simulink model "TrajectoryFollowVehicleWith14DoF_"  (R2024b)
settings: Solver=VariableStepAuto  StartTime=0  StopTime=14  FixedStep=timeStep  RelTol=1e-3
PreLoadFcn:
  | useDynamicsStanley = false; %Simulink model to move according to the scenario trajectory.
  | vehicleVariant = "3DOF";
PostLoadFcn:
  | load(fullfile(matlabroot,'toolbox','driving','drivingdata','rrScenarioSimTypes.mat'));
  | helperSLTrajectoryFollowerWithRRScenarioSetup();
  | hegihtMap = "flat";
  | if isfile("pathFollowingUtil/gridMap_groundHeight_RT.mat")
  |     load("gridMap_groundHeight_RT.mat");
  | end
  | % if exist("z_2DTable", "var") && exist("xBreakPts", "var") && exist("yBreakPts", "var")
  | %     hegihtMap = "2DMap";
  | % end
  | % if isfile("CRG/crgRoad.crg")
  | %     crgData = crg_read('CRG/crgRoad.crg');
  | % end
InitFcn:
  | if ~exist("slBus42", "var")
  |     load("Bus_VehFdbk.mat");
  | end
StartFcn:
  | % set_param(bdroot, 'Profile', 'on');
StopFcn:
  | % set_param(bdroot, 'Profile', 'off');
  | % slprofreport(bdroot, 'report14DoF.html');
undefined symbols (not defined in the file or in its folder): control_timeStep, Defined, Ego, egoInitialPose, egoInitialPoseCG, egoInitialPoseRear, InitVehicle, Lane, lr, m, magnitude, max_dc, n, Pose, RRtimeStep, SceneData, steerGear, tau, tau2, timeStep, User, VehicleData, Velocity, X, xBreakPts, Y, yBreakPts, Z, z_2DTable
libraries: sm_lib x40, nesl_utility x25, simulink_extras x12, sm_vehicle_utilities_lib x7, roadrunnerscenario x6, drivingvehiclecontroller x4, mpcadaslib x1, autolibshared x1
(part 3 of 3)

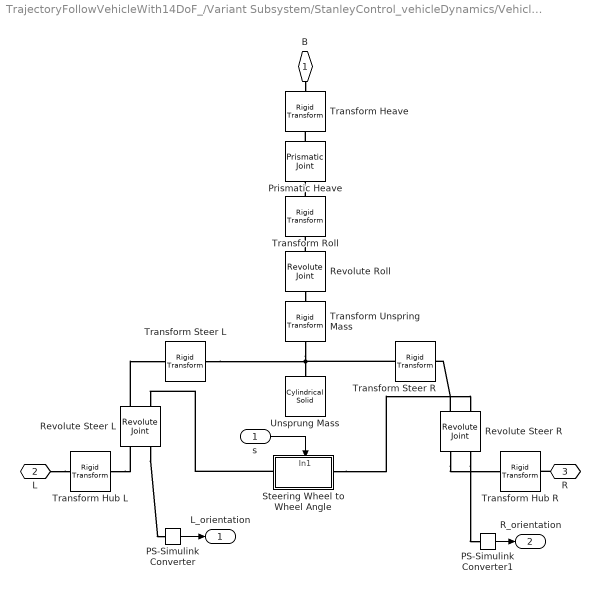
== system TrajectoryFollowVehicleWith14DoF_/Variant Subsystem/StanleyControl_vehicleDynamics/Vehicle Dynamics1/Vehicle Dynamics Multibody/Vehicle/Suspension Front ==
  s : Inport
  PS-Simulink Converter : nesl_utility/PS-Simulink Converter  PhysicalDomain=network_engine_domain  SubClassName=ps_output  LeftPortType=input  RightPortType=output  PseudoPeriodic=off  Frequencies=[]  VectorFormat=inherit  Unit=inherit  AffineConversion=off
  PS-Simulink Converter1 : nesl_utility/PS-Simulink Converter  PhysicalDomain=network_engine_domain  SubClassName=ps_output  LeftPortType=input  RightPortType=output  PseudoPeriodic=off  Frequencies=[]  VectorFormat=inherit  Unit=inherit  AffineConversion=off
  Prismatic Heave : sm_lib/Joints/Prismatic Joint  JointMode=Normal  CompositeWrenchDir=FollowerOnBase  CompositeWrenchFrame=BaseFrame  SenseConstraintForce=off  SenseConstraintTorque=off  SenseTotalForce=off  SenseTotalTorque=off  PositionTargetSpecify=off  PositionTargetPriority=High  PositionTargetValue=0  PositionTargetValueUnits=m  VelocityTargetSpecify=off  VelocityTargetPriority=High  VelocityTargetValue=0  VelocityTargetValueUnits=m/s  EquilibriumPosition=xEqHeave  EquilibriumPositionUnits=m  SpringStiffness=kHeave  SpringStiffnessUnits=N/m  DampingCoefficient=dHeave  DampingCoefficientUnits=N/(m/s)  LowerLimitSpecify=off  LowerLimitBound=-1  LowerLimitBoundUnits=m  LowerLimitStiffness=1e6  LowerLimitStiffnessUnits=N/m  LowerLimitDamping=1e3  LowerLimitDampingUnits=N/(m/s)  LowerLimitTransitionRegionWidth=1e-4  LowerLimitTransitionRegionWidthUnits=m  UpperLimitSpecify=off  UpperLimitBound=1  UpperLimitBoundUnits=m  UpperLimitStiffness=1e6  UpperLimitStiffnessUnits=N/m  UpperLimitDamping=1e3  UpperLimitDampingUnits=N/(m/s)  UpperLimitTransitionRegionWidth=1e-4  UpperLimitTransitionRegionWidthUnits=m  TorqueActuationMode=NoTorque  MotionActuationMode=ComputedMotion  SensePosition=off  SenseVelocity=off  SenseAcceleration=off  SenseTorqueForce=off  SenseLowerLimitTorqueForce=off  SenseUpperLimitTorqueForce=off
  Revolute Steer L : sm_lib/Joints/Revolute Joint  JointMode=Normal  CompositeWrenchDir=FollowerOnBase  CompositeWrenchFrame=BaseFrame  SenseConstraintForce=off  SenseConstraintTorque=off  SenseTotalForce=off  SenseTotalTorque=off  PositionTargetSpecify=off  PositionTargetPriority=High  PositionTargetValue=0  PositionTargetValueUnits=deg  VelocityTargetSpecify=off  VelocityTargetPriority=High  VelocityTargetValue=66  VelocityTargetValueUnits=rad/s  EquilibriumPosition=0  EquilibriumPositionUnits=rad  SpringStiffness=0  SpringStiffnessUnits=N*m/rad  DampingCoefficient=0  DampingCoefficientUnits=N*m/(rad/s)  LowerLimitSpecify=off  LowerLimitBound=-90  LowerLimitBoundUnits=deg  LowerLimitStiffness=1e4  LowerLimitStiffnessUnits=N*m/deg  LowerLimitDamping=10  LowerLimitDampingUnits=N*m/(deg/s)  LowerLimitTransitionRegionWidth=0.1  LowerLimitTransitionRegionWidthUnits=deg  UpperLimitSpecify=off  UpperLimitBound=90  UpperLimitBoundUnits=deg  UpperLimitStiffness=1e4  UpperLimitStiffnessUnits=N*m/deg  UpperLimitDamping=10  UpperLimitDampingUnits=N*m/(deg/s)  UpperLimitTransitionRegionWidth=0.1  UpperLimitTransitionRegionWidthUnits=deg  TorqueActuationMode=ComputedTorque  MotionActuationMode=InputMotion  SensePosition=on  SenseVelocity=off  SenseAcceleration=off  SenseTorqueForce=off  SenseLowerLimitTorqueForce=off  SenseUpperLimitTorqueForce=off
  Revolute Steer R : sm_lib/Joints/Revolute Joint  JointMode=Normal  CompositeWrenchDir=FollowerOnBase  CompositeWrenchFrame=BaseFrame  SenseConstraintForce=off  SenseConstraintTorque=off  SenseTotalForce=off  SenseTotalTorque=off  PositionTargetSpecify=off  PositionTargetPriority=High  PositionTargetValue=0  PositionTargetValueUnits=deg  VelocityTargetSpecify=off  VelocityTargetPriority=High  VelocityTargetValue=66  VelocityTargetValueUnits=rad/s  EquilibriumPosition=0  EquilibriumPositionUnits=rad  SpringStiffness=0  SpringStiffnessUnits=N*m/rad  DampingCoefficient=0  DampingCoefficientUnits=N*m/(rad/s)  LowerLimitSpecify=off  LowerLimitBound=-90  LowerLimitBoundUnits=deg  LowerLimitStiffness=1e4  LowerLimitStiffnessUnits=N*m/deg  LowerLimitDamping=10  LowerLimitDampingUnits=N*m/(deg/s)  LowerLimitTransitionRegionWidth=0.1  LowerLimitTransitionRegionWidthUnits=deg  UpperLimitSpecify=off  UpperLimitBound=90  UpperLimitBoundUnits=deg  UpperLimitStiffness=1e4  UpperLimitStiffnessUnits=N*m/deg  UpperLimitDamping=10  UpperLimitDampingUnits=N*m/(deg/s)  UpperLimitTransitionRegionWidth=0.1  UpperLimitTransitionRegionWidthUnits=deg  TorqueActuationMode=ComputedTorque  MotionActuationMode=InputMotion  SensePosition=on  SenseVelocity=off  SenseAcceleration=off  SenseTorqueForce=off  SenseLowerLimitTorqueForce=off  SenseUpperLimitTorqueForce=off
  Revolute Roll : sm_lib/Joints/Revolute Joint  JointMode=Normal  CompositeWrenchDir=FollowerOnBase  CompositeWrenchFrame=BaseFrame  SenseConstraintForce=off  SenseConstraintTorque=off  SenseTotalForce=off  SenseTotalTorque=off  PositionTargetSpecify=off  PositionTargetPriority=High  PositionTargetValue=0  PositionTargetValueUnits=deg  VelocityTargetSpecify=off  VelocityTargetPriority=High  VelocityTargetValue=0  VelocityTargetValueUnits=deg/s  EquilibriumPosition=aEqRoll  EquilibriumPositionUnits=rad  SpringStiffness=kRoll  SpringStiffnessUnits=N*m/rad  DampingCoefficient=dRoll  DampingCoefficientUnits=N*m/(rad/s)  LowerLimitSpecify=off  LowerLimitBound=-90  LowerLimitBoundUnits=deg  LowerLimitStiffness=1e4  LowerLimitStiffnessUnits=N*m/deg  LowerLimitDamping=10  LowerLimitDampingUnits=N*m/(deg/s)  LowerLimitTransitionRegionWidth=0.1  LowerLimitTransitionRegionWidthUnits=deg  UpperLimitSpecify=off  UpperLimitBound=90  UpperLimitBoundUnits=deg  UpperLimitStiffness=1e4  UpperLimitStiffnessUnits=N*m/deg  UpperLimitDamping=10  UpperLimitDampingUnits=N*m/(deg/s)  UpperLimitTransitionRegionWidth=0.1  UpperLimitTransitionRegionWidthUnits=deg  TorqueActuationMode=NoTorque  MotionActuationMode=ComputedMotion  SensePosition=off  SenseVelocity=off  SenseAcceleration=off  SenseTorqueForce=off  SenseLowerLimitTorqueForce=off  SenseUpperLimitTorqueForce=off
  Steering Wheel to Wheel Angle : Subsystem
      settings: PortSchema="{\"entries\":[{\"content\":{\"sides\":[{\"content\":{\"connectorIds\":[\"LConn1\"]},\"type\":\"ConnectorPlacement.EquallySpacedRectSide\",\"uuid\":\"65a6d75a-79bf-476b-9435-04bcf6c2ef18\"},{\"content\":{\"connectorIds\":[\"RConn1\"],\"side\":\"RIGHT\"},\"type\":\"ConnectorPlacement.EquallySpacedRectSide\",\"uuid\":\"4d91bb65-021e-4e19-8917-9509e9fd2683\"},{\"content\":{\"connectorIds\":[\"In1\"],\"side\":\"TOP\"},\"type\":\"ConnectorPlacement.EquallySpacedRectSide\",\"uuid\":\"f7aac0ed-f2d6-4a01-9627-e78393360ed0\"}]},\"type\":\"ConnectorPlacement.EquallySpacedConnector\",\"uuid\":\"6c2d29d9-099e-4079-9b4f-de2c4ae6c2a7\"}],\"packageUris\":[\"http://schema.mathworks.com/mf0/Connector/R2020b\"],\"version\":\"1.0\"}"
  Transform Heave : sm_lib/Frames and Transforms/Rigid Transform  RotationMethod=None  FollAlignAxisA=+X  BaseAlignAxisA=+Y  FollAlignAxisB=+Y  BaseAlignAxisB=+Z  RotationStandardAxis=+Z  RotationAngle=0.0  RotationAngleUnits=deg  RotationArbitraryAxis=[0 0 1]  RotationSequenceAxes=FollowerAxes  RotationSequence=XYX  RotationSequenceAngles=[0 0 0]  RotationSequenceAnglesUnits=deg  RotationMatrix=[1 0 0; 0 1 0; 0 0 1]  Quaternion=[1 0 0 0]  TranslationMethod=StandardAxis  TranslationCartesianOffset=[0 0 0]  TranslationCartesianOffsetUnits=m  TranslationStandardAxis=+Z  TranslationStandardOffset=zHeave  TranslationStandardOffsetUnits=m  TranslationROffset=0  TranslationROffsetUnits=m  TranslationThetaOffset=0  TranslationThetaOffsetUnits=deg  TranslationZOffset=0  TranslationZOffsetUnits=m
  Transform Hub L : sm_lib/Frames and Transforms/Rigid Transform  RotationMethod=StandardAxis  FollAlignAxisA=+X  BaseAlignAxisA=+Y  FollAlignAxisB=+Y  BaseAlignAxisB=+Z  RotationStandardAxis=-Y  RotationAngle=90  RotationAngleUnits=deg  RotationArbitraryAxis=[0 0 1]  RotationSequenceAxes=FollowerAxes  RotationSequence=XYX  RotationSequenceAngles=[0 0 0]  RotationSequenceAnglesUnits=deg  RotationMatrix=[1 0 0; 0 1 0; 0 0 1]  Quaternion=[1 0 0 0]  TranslationMethod=None  TranslationCartesianOffset=[0 0 0]  TranslationCartesianOffsetUnits=m  TranslationStandardAxis=+Z  TranslationStandardOffset=0  TranslationStandardOffsetUnits=m  TranslationROffset=0  TranslationROffsetUnits=m  TranslationThetaOffset=0  TranslationThetaOffsetUnits=deg  TranslationZOffset=0  TranslationZOffsetUnits=m
  Transform Hub R : sm_lib/Frames and Transforms/Rigid Transform  RotationMethod=StandardAxis  FollAlignAxisA=+X  BaseAlignAxisA=+Y  FollAlignAxisB=+Y  BaseAlignAxisB=+Z  RotationStandardAxis=-Y  RotationAngle=90  RotationAngleUnits=deg  RotationArbitraryAxis=[0 0 1]  RotationSequenceAxes=FollowerAxes  RotationSequence=XYX  RotationSequenceAngles=[0 0 0]  RotationSequenceAnglesUnits=deg  RotationMatrix=[1 0 0; 0 1 0; 0 0 1]  Quaternion=[1 0 0 0]  TranslationMethod=None  TranslationCartesianOffset=[0 0 0]  TranslationCartesianOffsetUnits=m  TranslationStandardAxis=+Z  TranslationStandardOffset=0  TranslationStandardOffsetUnits=m  TranslationROffset=0  TranslationROffsetUnits=m  TranslationThetaOffset=0  TranslationThetaOffsetUnits=deg  TranslationZOffset=0  TranslationZOffsetUnits=m
  Transform Roll : sm_lib/Frames and Transforms/Rigid Transform  RotationMethod=RotationSequence  FollAlignAxisA=+X  BaseAlignAxisA=+Y  FollAlignAxisB=+Y  BaseAlignAxisB=+Z  RotationStandardAxis=+Y  RotationAngle=90  RotationAngleUnits=deg  RotationArbitraryAxis=[0 0 1]  RotationSequenceAxes=FollowerAxes  RotationSequence=YZY  RotationSequenceAngles=[90 180 0]  RotationSequenceAnglesUnits=deg  RotationMatrix=[1 0 0; 0 1 0; 0 0 1]  Quaternion=[1 0 0 0]  TranslationMethod=StandardAxis  TranslationCartesianOffset=[0 0 0]  TranslationCartesianOffsetUnits=m  TranslationStandardAxis=+Z  TranslationStandardOffset=-zHeave+zRoll  TranslationStandardOffsetUnits=m  TranslationROffset=0  TranslationROffsetUnits=m  TranslationThetaOffset=0  TranslationThetaOffsetUnits=deg  TranslationZOffset=0  TranslationZOffsetUnits=m
  Transform Steer L : sm_lib/Frames and Transforms/Rigid Transform  RotationMethod=StandardAxis  FollAlignAxisA=+X  BaseAlignAxisA=+Y  FollAlignAxisB=+Y  BaseAlignAxisB=+Z  RotationStandardAxis=+Y  RotationAngle=90  RotationAngleUnits=deg  RotationArbitraryAxis=[0 0 1]  RotationSequenceAxes=FollowerAxes  RotationSequence=XYX  RotationSequenceAngles=[0 0 0]  RotationSequenceAnglesUnits=deg  RotationMatrix=[1 0 0; 0 1 0; 0 0 1]  Quaternion=[1 0 0 0]  TranslationMethod=Cartesian  TranslationCartesianOffset=[-zUnsprungMass+zHub 0 yTrack/2]  TranslationCartesianOffsetUnits=m  TranslationStandardAxis=+Z  TranslationStandardOffset=0  TranslationStandardOffsetUnits=m  TranslationROffset=0  TranslationROffsetUnits=m  TranslationThetaOffset=0  TranslationThetaOffsetUnits=deg  TranslationZOffset=0  TranslationZOffsetUnits=m
  Transform Steer R : sm_lib/Frames and Transforms/Rigid Transform  RotationMethod=StandardAxis  FollAlignAxisA=+X  BaseAlignAxisA=+Y  FollAlignAxisB=+Y  BaseAlignAxisB=+Z  RotationStandardAxis=+Y  RotationAngle=90  RotationAngleUnits=deg  RotationArbitraryAxis=[0 0 1]  RotationSequenceAxes=FollowerAxes  RotationSequence=XYX  RotationSequenceAngles=[0 0 0]  RotationSequenceAnglesUnits=deg  RotationMatrix=[1 0 0; 0 1 0; 0 0 1]  Quaternion=[1 0 0 0]  TranslationMethod=Cartesian  TranslationCartesianOffset=[-zUnsprungMass+zHub 0 -yTrack/2]  TranslationCartesianOffsetUnits=m  TranslationStandardAxis=+Z  TranslationStandardOffset=0  TranslationStandardOffsetUnits=m  TranslationROffset=0  TranslationROffsetUnits=m  TranslationThetaOffset=0  TranslationThetaOffsetUnits=deg  TranslationZOffset=0  TranslationZOffsetUnits=m
  Transform Unspring Mass : sm_lib/Frames and Transforms/Rigid Transform  RotationMethod=StandardAxis  FollAlignAxisA=+X  BaseAlignAxisA=+Y  FollAlignAxisB=+Y  BaseAlignAxisB=+Z  RotationStandardAxis=+X  RotationAngle=90  RotationAngleUnits=deg  RotationArbitraryAxis=[0 0 1]  RotationSequenceAxes=FollowerAxes  RotationSequence=XYX  RotationSequenceAngles=[0 0 0]  RotationSequenceAnglesUnits=deg  RotationMatrix=[1 0 0; 0 1 0; 0 0 1]  Quaternion=[1 0 0 0]  TranslationMethod=StandardAxis  TranslationCartesianOffset=[0 0 0]  TranslationCartesianOffsetUnits=m  TranslationStandardAxis=+X  TranslationStandardOffset=-zRoll+zUnsprungMass  TranslationStandardOffsetUnits=m  TranslationROffset=0  TranslationROffsetUnits=m  TranslationThetaOffset=0  TranslationThetaOffsetUnits=deg  TranslationZOffset=0  TranslationZOffsetUnits=m
  Unsprung Mass : sm_lib/Body Elements/Cylindrical Solid  CylinderRadius=rUnsprungMass  CylinderRadiusUnits=m  CylinderLength=lUnsprungMass  CylinderLengthUnits=m  ExportEntireGeometry=off  InertiaType=Custom  BasedOnType=Density  Density=1000  DensityUnits=kg/(m^3)  Mass=mUnsprungMass  MassUnits=kg  CenterOfMass=[0 0 0]  CenterOfMassUnits=m  MomentsOfInertia=JUnsprungMass  MomentsOfInertiaUnits=kg*m^2  ProductsOfInertia=[0 0 0]  ProductsOfInertiaUnits=kg*m^2  GraphicType=FromGeometry  MarkerShape=Sphere  MarkerSize=10  GraphicVisPropType=SimpleVisualProperties  GraphicDiffuseColor=[0.6 0.6 0.6]  GraphicOpacity=1.0  GraphicSpecularColor=[0.5 0.5 0.5 1.0]  GraphicAmbientColor=[0.15 0.15 0.15 1.0]  GraphicEmissiveColor=[0.0 0.0 0.0 1.0]  GraphicShininess=75  DoExposeReferenceFrame=on  SerializedFrames=<Frames/>
  B : PMIOPort  Side=Left
  L : PMIOPort  Port=2  Side=Left
  R : PMIOPort  Port=3  Side=Right
  L_orientation : Outport
  R_orientation : Outport  Port=2
  wires:
  s/1 -> Steering Wheel to Wheel Angle/1(In1)
  PS-Simulink Converter/1 -> L_orientation/1
  PS-Simulink Converter1/1 -> R_orientation/1
  connections:
  Transform Roll/LConn1 -- Prismatic Heave/RConn1
  Revolute Roll/LConn1 -- Transform Unspring Mass/LConn1
  Prismatic Heave/LConn1 -- Transform Heave/RConn1
  Steering Wheel to Wheel Angle/LConn1 -- Revolute Steer L/LConn2
  Steering Wheel to Wheel Angle/RConn1 -- Revolute Steer R/LConn2
  B/RConn1 -- Transform Heave/LConn1
  Revolute Roll/RConn1 -- Transform Roll/RConn1
  L/RConn1 -- Transform Hub L/RConn1
  Transform Hub L/LConn1 -- Revolute Steer L/RConn1
  R/RConn1 -- Transform Hub R/RConn1
  Revolute Steer R/RConn1 -- Transform Hub R/LConn1
  Transform Steer L/LConn1 -- Transform Unspring Mass/RConn1 -- Transform Steer R/LConn1 -- Unsprung Mass/RConn1
  Revolute Steer R/LConn1 -- Transform Steer R/RConn1
  Revolute Steer L/LConn1 -- Transform Steer L/RConn1
  Revolute Steer L/RConn2 -- PS-Simulink Converter/LConn1
  Revolute Steer R/RConn2 -- PS-Simulink Converter1/LConn1

== system TrajectoryFollowVehicleWith14DoF_/Variant Subsystem/StanleyControl_vehicleDynamics/Vehicle Dynamics1/Vehicle Dynamics Multibody/Vehicle/Suspension Rear ==
  Prismatic Heave : sm_lib/Joints/Prismatic Joint  JointMode=Normal  CompositeWrenchDir=FollowerOnBase  CompositeWrenchFrame=BaseFrame  SenseConstraintForce=off  SenseConstraintTorque=off  SenseTotalForce=off  SenseTotalTorque=off  PositionTargetSpecify=off  PositionTargetPriority=High  PositionTargetValue=0  PositionTargetValueUnits=m  VelocityTargetSpecify=off  VelocityTargetPriority=High  VelocityTargetValue=0  VelocityTargetValueUnits=m/s  EquilibriumPosition=xEqHeave  EquilibriumPositionUnits=m  SpringStiffness=kHeave  SpringStiffnessUnits=N/m  DampingCoefficient=dHeave  DampingCoefficientUnits=N/(m/s)  LowerLimitSpecify=off  LowerLimitBound=-1  LowerLimitBoundUnits=m  LowerLimitStiffness=1e6  LowerLimitStiffnessUnits=N/m  LowerLimitDamping=1e3  LowerLimitDampingUnits=N/(m/s)  LowerLimitTransitionRegionWidth=1e-4  LowerLimitTransitionRegionWidthUnits=m  UpperLimitSpecify=off  UpperLimitBound=1  UpperLimitBoundUnits=m  UpperLimitStiffness=1e6  UpperLimitStiffnessUnits=N/m  UpperLimitDamping=1e3  UpperLimitDampingUnits=N/(m/s)  UpperLimitTransitionRegionWidth=1e-4  UpperLimitTransitionRegionWidthUnits=m  TorqueActuationMode=NoTorque  MotionActuationMode=ComputedMotion  SensePosition=off  SenseVelocity=off  SenseAcceleration=off  SenseTorqueForce=off  SenseLowerLimitTorqueForce=off  SenseUpperLimitTorqueForce=off
  Revolute Roll : sm_lib/Joints/Revolute Joint  JointMode=Normal  CompositeWrenchDir=FollowerOnBase  CompositeWrenchFrame=BaseFrame  SenseConstraintForce=off  SenseConstraintTorque=off  SenseTotalForce=off  SenseTotalTorque=off  PositionTargetSpecify=off  PositionTargetPriority=High  PositionTargetValue=0  PositionTargetValueUnits=deg  VelocityTargetSpecify=off  VelocityTargetPriority=High  VelocityTargetValue=0  VelocityTargetValueUnits=deg/s  EquilibriumPosition=aEqRoll  EquilibriumPositionUnits=rad  SpringStiffness=kRoll  SpringStiffnessUnits=N*m/rad  DampingCoefficient=dRoll  DampingCoefficientUnits=N*m/(rad/s)  LowerLimitSpecify=off  LowerLimitBound=-90  LowerLimitBoundUnits=deg  LowerLimitStiffness=1e4  LowerLimitStiffnessUnits=N*m/deg  LowerLimitDamping=10  LowerLimitDampingUnits=N*m/(deg/s)  LowerLimitTransitionRegionWidth=0.1  LowerLimitTransitionRegionWidthUnits=deg  UpperLimitSpecify=off  UpperLimitBound=90  UpperLimitBoundUnits=deg  UpperLimitStiffness=1e4  UpperLimitStiffnessUnits=N*m/deg  UpperLimitDamping=10  UpperLimitDampingUnits=N*m/(deg/s)  UpperLimitTransitionRegionWidth=0.1  UpperLimitTransitionRegionWidthUnits=deg  TorqueActuationMode=NoTorque  MotionActuationMode=ComputedMotion  SensePosition=off  SenseVelocity=off  SenseAcceleration=off  SenseTorqueForce=off  SenseLowerLimitTorqueForce=off  SenseUpperLimitTorqueForce=off
  Transform Heave : sm_lib/Frames and Transforms/Rigid Transform  RotationMethod=None  FollAlignAxisA=+X  BaseAlignAxisA=+Y  FollAlignAxisB=+Y  BaseAlignAxisB=+Z  RotationStandardAxis=+Z  RotationAngle=0.0  RotationAngleUnits=deg  RotationArbitraryAxis=[0 0 1]  RotationSequenceAxes=FollowerAxes  RotationSequence=XYX  RotationSequenceAngles=[0 0 0]  RotationSequenceAnglesUnits=deg  RotationMatrix=[1 0 0; 0 1 0; 0 0 1]  Quaternion=[1 0 0 0]  TranslationMethod=StandardAxis  TranslationCartesianOffset=[0 0 0]  TranslationCartesianOffsetUnits=m  TranslationStandardAxis=+Z  TranslationStandardOffset=zHeave  TranslationStandardOffsetUnits=m  TranslationROffset=0  TranslationROffsetUnits=m  TranslationThetaOffset=0  TranslationThetaOffsetUnits=deg  TranslationZOffset=0  TranslationZOffsetUnits=m
  Transform Hub L : sm_lib/Frames and Transforms/Rigid Transform  RotationMethod=None  FollAlignAxisA=+X  BaseAlignAxisA=+Y  FollAlignAxisB=+Y  BaseAlignAxisB=+Z  RotationStandardAxis=+X  RotationAngle=0  RotationAngleUnits=deg  RotationArbitraryAxis=[0 0 1]  RotationSequenceAxes=FollowerAxes  RotationSequence=XYX  RotationSequenceAngles=[0 0 0]  RotationSequenceAnglesUnits=deg  RotationMatrix=[1 0 0; 0 1 0; 0 0 1]  Quaternion=[1 0 0 0]  TranslationMethod=Cartesian  TranslationCartesianOffset=[-zUnsprungMass+zHub 0 yTrack/2]  TranslationCartesianOffsetUnits=m  TranslationStandardAxis=+Z  TranslationStandardOffset=0  TranslationStandardOffsetUnits=m  TranslationROffset=0  TranslationROffsetUnits=m  TranslationThetaOffset=0  TranslationThetaOffsetUnits=deg  TranslationZOffset=0  TranslationZOffsetUnits=m
  Transform Hub R : sm_lib/Frames and Transforms/Rigid Transform  RotationMethod=None  FollAlignAxisA=+X  BaseAlignAxisA=+Y  FollAlignAxisB=+Y  BaseAlignAxisB=+Z  RotationStandardAxis=+X  RotationAngle=0  RotationAngleUnits=deg  RotationArbitraryAxis=[0 0 1]  RotationSequenceAxes=FollowerAxes  RotationSequence=XYX  RotationSequenceAngles=[0 0 0]  RotationSequenceAnglesUnits=deg  RotationMatrix=[1 0 0; 0 1 0; 0 0 1]  Quaternion=[1 0 0 0]  TranslationMethod=Cartesian  TranslationCartesianOffset=[-zUnsprungMass+zHub 0 -yTrack/2]  TranslationCartesianOffsetUnits=m  TranslationStandardAxis=+Z  TranslationStandardOffset=0  TranslationStandardOffsetUnits=m  TranslationROffset=0  TranslationROffsetUnits=m  TranslationThetaOffset=0  TranslationThetaOffsetUnits=deg  TranslationZOffset=0  TranslationZOffsetUnits=m
  Transform Roll : sm_lib/Frames and Transforms/Rigid Transform  RotationMethod=RotationSequence  FollAlignAxisA=+X  BaseAlignAxisA=+Y  FollAlignAxisB=+Y  BaseAlignAxisB=+Z  RotationStandardAxis=+Y  RotationAngle=90  RotationAngleUnits=deg  RotationArbitraryAxis=[0 0 1]  RotationSequenceAxes=FollowerAxes  RotationSequence=YZY  RotationSequenceAngles=[90 180 0]  RotationSequenceAnglesUnits=deg  RotationMatrix=[1 0 0; 0 1 0; 0 0 1]  Quaternion=[1 0 0 0]  TranslationMethod=StandardAxis  TranslationCartesianOffset=[0 0 0]  TranslationCartesianOffsetUnits=m  TranslationStandardAxis=+Z  TranslationStandardOffset=-zHeave+zRoll  TranslationStandardOffsetUnits=m  TranslationROffset=0  TranslationROffsetUnits=m  TranslationThetaOffset=0  TranslationThetaOffsetUnits=deg  TranslationZOffset=0  TranslationZOffsetUnits=m
  Transform Unsprung Mass : sm_lib/Frames and Transforms/Rigid Transform  RotationMethod=StandardAxis  FollAlignAxisA=+X  BaseAlignAxisA=+Y  FollAlignAxisB=+Y  BaseAlignAxisB=+Z  RotationStandardAxis=+X  RotationAngle=90  RotationAngleUnits=deg  RotationArbitraryAxis=[0 0 1]  RotationSequenceAxes=FollowerAxes  RotationSequence=XYX  RotationSequenceAngles=[0 0 0]  RotationSequenceAnglesUnits=deg  RotationMatrix=[1 0 0; 0 1 0; 0 0 1]  Quaternion=[1 0 0 0]  TranslationMethod=StandardAxis  TranslationCartesianOffset=[0 0 0]  TranslationCartesianOffsetUnits=m  TranslationStandardAxis=+X  TranslationStandardOffset=-zRoll+zUnsprungMass  TranslationStandardOffsetUnits=m  TranslationROffset=0  TranslationROffsetUnits=m  TranslationThetaOffset=0  TranslationThetaOffsetUnits=deg  TranslationZOffset=0  TranslationZOffsetUnits=m
  Unsprung Mass : sm_lib/Body Elements/Cylindrical Solid  CylinderRadius=rUnsprungMass  CylinderRadiusUnits=m  CylinderLength=lUnsprungMass  CylinderLengthUnits=m  ExportEntireGeometry=off  InertiaType=Custom  BasedOnType=Density  Density=1000  DensityUnits=kg/(m^3)  Mass=mUnsprungMass  MassUnits=kg  CenterOfMass=[0 0 0]  CenterOfMassUnits=m  MomentsOfInertia=JUnsprungMass  MomentsOfInertiaUnits=kg*m^2  ProductsOfInertia=[0 0 0]  ProductsOfInertiaUnits=kg*m^2  GraphicType=FromGeometry  MarkerShape=Sphere  MarkerSize=10  GraphicVisPropType=SimpleVisualProperties  GraphicDiffuseColor=[0.6 0.6 0.6]  GraphicOpacity=1.0  GraphicSpecularColor=[0.5 0.5 0.5 1.0]  GraphicAmbientColor=[0.15 0.15 0.15 1.0]  GraphicEmissiveColor=[0.0 0.0 0.0 1.0]  GraphicShininess=75  DoExposeReferenceFrame=on  SerializedFrames=<Frames/>
  B : PMIOPort  Side=Left
  L : PMIOPort  Port=2  Side=Left
  R : PMIOPort  Port=3  Side=Right
  connections:
  Revolute Roll/RConn1 -- Transform Roll/RConn1
  Transform Roll/LConn1 -- Prismatic Heave/RConn1
  Transform Hub R/RConn1 -- R/RConn1
  Transform Heave/LConn1 -- B/RConn1
  Transform Heave/RConn1 -- Prismatic Heave/LConn1
  L/RConn1 -- Transform Hub L/RConn1
  Revolute Roll/LConn1 -- Transform Unsprung Mass/LConn1
  Unsprung Mass/RConn1 -- Transform Hub R/LConn1 -- Transform Hub L/LConn1 -- Transform Unsprung Mass/RConn1

== system TrajectoryFollowVehicleWith14DoF_/Variant Subsystem/StanleyControl_vehicleDynamics/Vehicle Dynamics1/Vehicle Dynamics Multibody/Vehicle/World ==
  Mechanism Configuration : sm_lib/Utilities/Mechanism Configuration  UniformGravity=Constant  GravityVector=[0 0 -10]  GravityVectorUnits=m/s^2  LinearizationDelta=0.001  JointModeTransitionNonlinearIterations=2
  Solver Configuration : nesl_utility/Solver Configuration  PhysicalDomain=network_engine_domain  SubClassName=solver  LeftPortType=input  RightPortType=generic  Tones=[]  Harmonics=[]  SimulateNoise=off  Profile=off  UseLocalSampling=off  EnableSwitchedLinearOptims=on  FrequencyDomain=off  UseCCode=off  RelTol=0.001  AbsTol=1e-06  MinStep=1e-09  ToWorkspace=off  RevertToSquareIcSolve=off  NumHomotopyIterations=100  PhasorMode=off  PhasorModeNumHarmonics=1  ConsistencySolver=NEWTON_FTOL  IndexReductionMethod=DerivativeReplacement  DoDC=off  ResidualTolerance=1e-9  ConsistencyTolSource=GLOBAL  ConsistencyAbsTol=0.001  ConsistencyRelTol=0.001  ConsistencyTolFactor=0.001  UseLocalSolver=off  LocalSolverChoice=NE_BACKWARD_EULER_ADVANCER  ResolveIndetEquations=on  FunctionEvalNumThread=1  LocalSolverSampleTime=.001  DoFixedCost=off  MaxNonlinIter=3  MaxModeIter=2  ComputeImpulses=off  ImpulseIterations=2  LinearAlgebra=Sparse  LinearAlgebraNumThread=0  EquationFormulation=NE_TIME_EF  DelaysMemoryBudget=1024  AutomaticFiltering=on  FilteringTimeConstant=0.001  PartitionStorageMethod=AS_NEEDED  PartitionMemoryBudget=1024  PartitionMethod=FAST  MultibodyUseLocalSolver=off  MultibodyLocalSolverChoice=ODE1  MultibodyLocalSolverSampleTime=0.001
  World Frame : sm_lib/Frames and Transforms/World Frame
  W : PMIOPort  Side=Right
  connections:
  Solver Configuration/RConn1 -- World Frame/RConn1 -- W/RConn1 -- Mechanism Configuration/RConn1

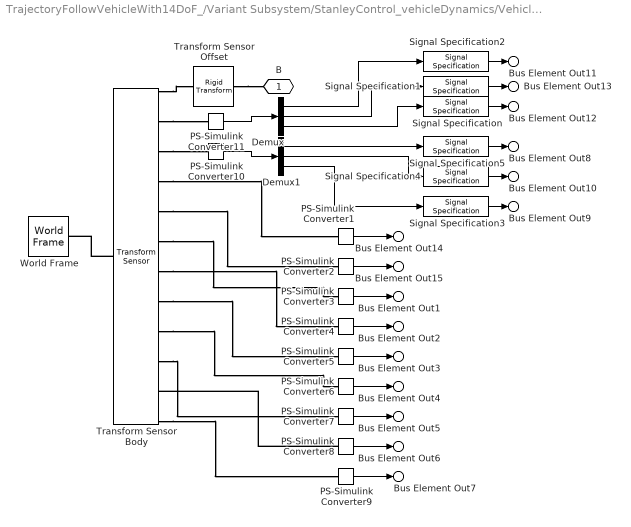
== system TrajectoryFollowVehicleWith14DoF_/Variant Subsystem/StanleyControl_vehicleDynamics/Vehicle Dynamics1/Vehicle Dynamics Multibody/Vehicle/Body/MyBodySensor ==
  Demux : Demux  Outputs=3
  Demux1 : Demux  Outputs=3
  PS-Simulink Converter1 : nesl_utility/PS-Simulink Converter  PhysicalDomain=network_engine_domain  SubClassName=ps_output  LeftPortType=input  RightPortType=output  PseudoPeriodic=off  Frequencies=[]  VectorFormat=1-D array  Unit=m  AffineConversion=off
  PS-Simulink Converter10 : nesl_utility/PS-Simulink Converter  PhysicalDomain=network_engine_domain  SubClassName=ps_output  LeftPortType=input  RightPortType=output  PseudoPeriodic=off  Frequencies=[]  VectorFormat=1-D array  Unit=rad/s  AffineConversion=off
  PS-Simulink Converter11 : nesl_utility/PS-Simulink Converter  PhysicalDomain=network_engine_domain  SubClassName=ps_output  LeftPortType=input  RightPortType=output  PseudoPeriodic=off  Frequencies=[]  VectorFormat=1-D array  Unit=rad  AffineConversion=off
  PS-Simulink Converter2 : nesl_utility/PS-Simulink Converter  PhysicalDomain=network_engine_domain  SubClassName=ps_output  LeftPortType=input  RightPortType=output  PseudoPeriodic=off  Frequencies=[]  VectorFormat=1-D array  Unit=m  AffineConversion=off
  PS-Simulink Converter3 : nesl_utility/PS-Simulink Converter  PhysicalDomain=network_engine_domain  SubClassName=ps_output  LeftPortType=input  RightPortType=output  PseudoPeriodic=off  Frequencies=[]  VectorFormat=1-D array  Unit=m  AffineConversion=off
  PS-Simulink Converter4 : nesl_utility/PS-Simulink Converter  PhysicalDomain=network_engine_domain  SubClassName=ps_output  LeftPortType=input  RightPortType=output  PseudoPeriodic=off  Frequencies=[]  VectorFormat=1-D array  Unit=m/s  AffineConversion=off
  PS-Simulink Converter5 : nesl_utility/PS-Simulink Converter  PhysicalDomain=network_engine_domain  SubClassName=ps_output  LeftPortType=input  RightPortType=output  PseudoPeriodic=off  Frequencies=[]  VectorFormat=1-D array  Unit=m/s  AffineConversion=off
  PS-Simulink Converter6 : nesl_utility/PS-Simulink Converter  PhysicalDomain=network_engine_domain  SubClassName=ps_output  LeftPortType=input  RightPortType=output  PseudoPeriodic=off  Frequencies=[]  VectorFormat=1-D array  Unit=m/s  AffineConversion=off
  PS-Simulink Converter7 : nesl_utility/PS-Simulink Converter  PhysicalDomain=network_engine_domain  SubClassName=ps_output  LeftPortType=input  RightPortType=output  PseudoPeriodic=off  Frequencies=[]  VectorFormat=1-D array  Unit=m/s^2  AffineConversion=off
  PS-Simulink Converter8 : nesl_utility/PS-Simulink Converter  PhysicalDomain=network_engine_domain  SubClassName=ps_output  LeftPortType=input  RightPortType=output  PseudoPeriodic=off  Frequencies=[]  VectorFormat=1-D array  Unit=m/s^2  AffineConversion=off
  PS-Simulink Converter9 : nesl_utility/PS-Simulink Converter  PhysicalDomain=network_engine_domain  SubClassName=ps_output  LeftPortType=input  RightPortType=output  PseudoPeriodic=off  Frequencies=[]  VectorFormat=1-D array  Unit=m/s^2  AffineConversion=off
  Signal Specification : SignalSpecification  Unit=rad
  Signal Specification1 : SignalSpecification  Unit=rad
  Signal Specification2 : SignalSpecification  Unit=rad
  Signal Specification3 : SignalSpecification  Unit=rad/s
  Signal Specification4 : SignalSpecification  Unit=rad/s
  Signal Specification5 : SignalSpecification  Unit=rad/s
  Transform Sensor Offset : sm_lib/Frames and Transforms/Rigid Transform  RotationMethod=None  FollAlignAxisA=+X  BaseAlignAxisA=+Y  FollAlignAxisB=+Y  BaseAlignAxisB=+Z  RotationStandardAxis=+Z  RotationAngle=0.0  RotationAngleUnits=deg  RotationArbitraryAxis=[0 0 1]  RotationSequenceAxes=FollowerAxes  RotationSequence=XYX  RotationSequenceAngles=[0 0 0]  RotationSequenceAnglesUnits=deg  RotationMatrix=[1 0 0; 0 1 0; 0 0 1]  Quaternion=[1 0 0 0]  TranslationMethod=Cartesian  TranslationCartesianOffset=[0, 0, 0]  TranslationCartesianOffsetUnits=m  TranslationStandardAxis=+Z  TranslationStandardOffset=0  TranslationStandardOffsetUnits=m  TranslationROffset=0  TranslationROffsetUnits=m  TranslationThetaOffset=0  TranslationThetaOffsetUnits=deg  TranslationZOffset=0  TranslationZOffsetUnits=m
  Transform Sensor Body : sm_lib/Frames and Transforms/Transform Sensor  MeasurementFrame=World  RotationSequence=ZYX  SenseAngle=off  SenseAxis=off  SenseQ=off  SenseR=off  SenseRotationSequence=on  SenseOmegaX=off  SenseOmegaY=off  SenseOmegaZ=off  SenseOmega=on  SenseQDot=off  SenseRDot=off  SenseRotationSequenceDot=off  SenseAlphaX=off  SenseAlphaY=off  SenseAlphaZ=off  SenseAlpha=off  SenseQDDot=off  SenseRDDot=off  SenseX=on  SenseY=on  SenseZ=on  SenseXYZ=off  SenseRad=off  SenseAzim=off  SenseDist=off  SenseInc=off  SenseXDot=on  SenseYDot=on  SenseZDot=on  SenseXYZDot=off  SenseRadDot=off  SenseAzimDot=off  SenseDistDot=off  SenseIncDot=off  SenseXDDot=on  SenseYDDot=on  SenseZDDot=on  SenseXYZDDot=off  SenseRadDDot=off  SenseAzimDDot=off  SenseDistDDot=off  SenseIncDDot=off
  World Frame : sm_lib/Frames and Transforms/World Frame
  B : PMIOPort  Side=Left
  Bus Element Out9 : Outport  VectorParamsAs1DForOutWhenUnconnected=off  PortName=Body  Element=nRoll
  Bus Element Out10 : Outport  VectorParamsAs1DForOutWhenUnconnected=off  PortName=Body  Element=nPitch
  Bus Element Out12 : Outport  VectorParamsAs1DForOutWhenUnconnected=off  PortName=Body  Element=aRoll
  Bus Element Out13 : Outport  VectorParamsAs1DForOutWhenUnconnected=off  PortName=Body  Element=aPitch
  Bus Element Out11 : Outport  VectorParamsAs1DForOutWhenUnconnected=off  PortName=Body  Element=aYaw
  Bus Element Out14 : Outport  VectorParamsAs1DForOutWhenUnconnected=off  PortName=Body  Element=x
  Bus Element Out15 : Outport  VectorParamsAs1DForOutWhenUnconnected=off  PortName=Body  Element=y
  Bus Element Out1 : Outport  VectorParamsAs1DForOutWhenUnconnected=off  PortName=Body  Element=z
  Bus Element Out2 : Outport  VectorParamsAs1DForOutWhenUnconnected=off  PortName=Body  Element=vx
  Bus Element Out3 : Outport  VectorParamsAs1DForOutWhenUnconnected=off  PortName=Body  Element=vy
  Bus Element Out4 : Outport  VectorParamsAs1DForOutWhenUnconnected=off  PortName=Body  Element=vz
  Bus Element Out5 : Outport  VectorParamsAs1DForOutWhenUnconnected=off  PortName=Body  Element=gx
  Bus Element Out6 : Outport  VectorParamsAs1DForOutWhenUnconnected=off  PortName=Body  Element=gy
  Bus Element Out7 : Outport  VectorParamsAs1DForOutWhenUnconnected=off  PortName=Body  Element=gz
  Bus Element Out8 : Outport  VectorParamsAs1DForOutWhenUnconnected=off  PortName=Body  Element=nYaw
  wires:
  Demux1/2 -> Signal Specification4/1
  Signal Specification1/1 -> Bus Element Out13/1
  Demux/2 -> Signal Specification1/1
  Signal Specification4/1 -> Bus Element Out10/1
  Demux/3 -> Signal Specification/1
  Signal Specification/1 -> Bus Element Out12/1
  Demux1/3 -> Signal Specification3/1
  PS-Simulink Converter11/1 -> Demux/1
  Signal Specification3/1 -> Bus Element Out9/1
  PS-Simulink Converter9/1 -> Bus Element Out7/1
  PS-Simulink Converter2/1 -> Bus Element Out15/1
  PS-Simulink Converter3/1 -> Bus Element Out1/1
  PS-Simulink Converter4/1 -> Bus Element Out2/1
  PS-Simulink Converter1/1 -> Bus Element Out14/1
  PS-Simulink Converter8/1 -> Bus Element Out6/1
  PS-Simulink Converter5/1 -> Bus Element Out3/1
  PS-Simulink Converter6/1 -> Bus Element Out4/1
  PS-Simulink Converter7/1 -> Bus Element Out5/1
  Demux/1 -> Signal Specification2/1
  Signal Specification2/1 -> Bus Element Out11/1
  PS-Simulink Converter10/1 -> Demux1/1
  Signal Specification5/1 -> Bus Element Out8/1
  Demux1/1 -> Signal Specification5/1
  connections:
  Transform Sensor Body/RConn7 -- PS-Simulink Converter4/LConn1
  Transform Sensor Body/RConn1 -- Transform Sensor Offset/RConn1
  Transform Sensor Body/RConn2 -- PS-Simulink Converter11/LConn1
  PS-Simulink Converter8/LConn1 -- Transform Sensor Body/RConn11
  Transform Sensor Body/RConn6 -- PS-Simulink Converter3/LConn1
  Transform Sensor Body/RConn8 -- PS-Simulink Converter5/LConn1
  Transform Sensor Offset/LConn1 -- B/RConn1
  Transform Sensor Body/RConn4 -- PS-Simulink Converter1/LConn1
  Transform Sensor Body/RConn9 -- PS-Simulink Converter6/LConn1
  Transform Sensor Body/LConn1 -- World Frame/RConn1
  Transform Sensor Body/RConn10 -- PS-Simulink Converter7/LConn1
  Transform Sensor Body/RConn5 -- PS-Simulink Converter2/LConn1
  Transform Sensor Body/RConn3 -- PS-Simulink Converter10/LConn1
  Transform Sensor Body/RConn12 -- PS-Simulink Converter9/LConn1

== system TrajectoryFollowVehicleWith14DoF_/Variant Subsystem/StanleyControl_vehicleDynamics/Vehicle Dynamics1/Vehicle Dynamics Multibody/Vehicle/Suspension Front/Steering Wheel to Wheel Angle ==
  In1 : Inport
  Ackerman left : Fcn  Expr=atan( 1/( cos(u+eps)/sin(u+eps) - yTrack/(2*wheelbase) ) )
  Ackerman right : Fcn  Expr=atan( 1/( cos(u+eps)/sin(u+eps) + yTrack/(2*wheelbase) ) )
  Constant : Constant  Value=steerRatio
  Divide : Product  Inputs=*/
  Simulink-PS Converter : nesl_utility/Simulink-PS Converter  PhysicalDomain=network_engine_domain  SubClassName=ps_input  LeftPortType=input  RightPortType=output  PseudoPeriodic=off  Frequencies=[]  NoiseDistribution=none  NoiseParameters=[]  Unit=rad  AffineConversion=off  FilteringAndDerivatives=filter  SimscapeFilterOrder=2  InputFilterTimeConstant=0.0055  UdotUserProvided=2
  Simulink-PS Converter1 : nesl_utility/Simulink-PS Converter  PhysicalDomain=network_engine_domain  SubClassName=ps_input  LeftPortType=input  RightPortType=output  PseudoPeriodic=off  Frequencies=[]  NoiseDistribution=none  NoiseParameters=[]  Unit=rad  AffineConversion=off  FilteringAndDerivatives=filter  SimscapeFilterOrder=2  InputFilterTimeConstant=0.0055  UdotUserProvided=2
  L : PMIOPort  Side=Left
  R : PMIOPort  Port=2  Side=Right
  wires:
  In1/1 -> Divide/1
  Ackerman left/1 -> Simulink-PS Converter1/1
  Ackerman right/1 -> Simulink-PS Converter/1
  Constant/1 -> Divide/2
  Divide/1 -> Ackerman right/1, Ackerman left/1
  connections:
  Simulink-PS Converter/RConn1 -- R/RConn1
  Simulink-PS Converter1/RConn1 -- L/RConn1

== matlab function TrajectoryFollowVehicleWith14DoF_/Pack Actor Pose/Pose Generation ==
  data: pose input; currPose output
function currPose = generatePose(pose)
% pose = [x y yaw_rad z pitch_rad]
yaw = deg2rad(pose(3));
pitch = deg2rad(pose(5));
roll = deg2rad(pose(6));
rotm = eul2rotm([yaw pitch roll], "ZYX");

currPose = [[rotm [pose([1 2 4])]']; [0 0 0 1]];

== matlab function TrajectoryFollowVehicleWith14DoF_/Variant Subsystem/StanleyControl_vehicleDynamics/Variant Subsystem/MPC/MATLAB Function ==
  data: u input; y output; offset input
function y = fcn(u, offset)
% u: x y yaw_deg z pitch 

y = u(1, :);
rotm = eul2rotm(deg2rad([u(1, 3), u(1, 5), 0]), "ZYX");
offset_3d = rotm * [offset; 0; 0];

y([1, 2, 4]) = u(1, [1, 2, 4]) + offset_3d';

== matlab function TrajectoryFollowVehicleWith14DoF_/Pack Actor Pose/Velocity XYZ Components ==
  data: yaw_pitch input size=2; velocity output size=[1 3]; speed input size=1
function velocity = computeVelocity(yaw_pitch, speed)

% Output velocity vector (x,y,z)
yaw = yaw_pitch(1);
pitch = yaw_pitch(2);
xyVel = speed * cosd(pitch);
zVel = speed * -sind(pitch);
velocity = [xyVel * cosd(yaw), xyVel * sind(yaw), zVel];

== matlab function TrajectoryFollowVehicleWith14DoF_/Variant Subsystem/StanleyControl_vehicleDynamics/Vehicle Dynamics1/Vehicle Dynamics Multibody/mean ==
  data: u input; y output
function y = fcn(u)
y = (u(1) + u(2)) / 2.0;

== matlab function TrajectoryFollowVehicleWith14DoF_/Variant Subsystem/StanleyControl_vehicleDynamics/Lateral Metrics ==
  data: currPose input size=[1 3]; refPose input size=[1 3]; positionError output; headingError output
function [positionError, headingError] = lateralMetrics(currPose, refPose)
%lateralMetrics calculates lateral error and heading error of the vehicle 
% using current and reference pose

currPose(:,3) = deg2rad(currPose(:,3));
refPose(:,3)  = deg2rad(refPose(:,3));

positionError = norm(currPose(1:2) - refPose(1:2));

headingError = rad2deg(currPose(:, 3) - refPose(:,3));

== matlab function TrajectoryFollowVehicleWith14DoF_/Variant Subsystem/StanleyControl_vehicleDynamics/Variant Subsystem/MPC/MATLAB Function1 ==
  data: u input; y output; offset input
function y = fcn(u, offset)
% u: x y yaw_deg z pitch 

y = u;
rotm = eul2rotm(deg2rad([u(3), u(5), 0]), "ZYX");
offset_3d = rotm * [offset; 0; 0];

y([1, 2, 4]) = u([1, 2, 4]) + offset_3d';

== matlab function TrajectoryFollowVehicleWith14DoF_/Variant Subsystem/StanleyControl_vehicleDynamics/Variant Subsystem/MPC/MATLAB Function2 ==
  data: refPose input; lateral_deviation output; currPose input; yaw_diff_rad output
function [lateral_deviation, yaw_diff_rad] = fcn(refPose, currPose)
% lateral deviation
% Ego vehicle lateral deviation in meters from the centerline of the lane.
% The lateral deviation e1 is positive when the ego vehicle is to the right of the centerline and negative when the ego vehicle is to the left of the centerline.
% yaw_diff
% Ego vehicle longitudinal axis angle in radians from the centerline of the lane, defined as:
% Here, θe is the ego vehicle angle and θc is the centerline angle, with both angles defined in the global coordinate frame.
% refYaw = deg2rad(refPose(3));
% rotm = [cos(refYaw), -sin(refYaw); sin(refYaw) cos(refYaw)];

yaw = deg2rad(currPose(3));
rotm = [cos(yaw), -sin(yaw); sin(yaw) cos(yaw)];
rotm_inv = transpose(rotm);

refXY = rotm_inv * refPose(1:2);
currXY = rotm_inv * currPose(1:2);

lateral_deviation = currXY(2) - refXY(2);
yaw_diff_rad = deg2rad(currPose(3) - refPose(3));
while yaw_diff_rad >= 2*pi
    yaw_diff_rad = yaw_diff_rad - 2*pi;
end
while yaw_diff_rad <= -2*pi
    yaw_diff_rad = yaw_diff_rad + 2*pi;
end

== matlab function TrajectoryFollowVehicleWith14DoF_/Variant Subsystem/StanleyControl_vehicleDynamics/Vehicle Dynamics1/Vehicle Dynamics 14DOF/Variant Subsystem/2DHeightMap/MATLAB Function ==
  data: x input; y input; z input
function debug2DTablePlot(x, y, z)
%#codegen
% 入力: x, y, z は [1×4] の double ベクトル
%       （4点分の x座標, y座標, z座標）
%
% この関数が最初に呼ばれた時に 2D Lookup Table の面を描画。
% 以降の呼び出しで (x,y,z) の4点を更新表示する。
 
% --- Simulink コード生成でグラフィックス関数は対象外なので 'extrinsic' 指定 ---
coder.extrinsic('evalin','figure','meshgrid','surf','colormap','shading','colorbar',...
                 'xlabel','ylabel','zlabel','title','hold','plot3','drawnow', 'set');
 
% --- 初期化済みかどうか判定するフラグ ---
persistent isInitialized  figH  lineH
 
if isempty(isInitialized)
    %============================
    % (A) 初回呼び出し時のみ、Figure の初期化＆Lookup Table の面を描画
    %============================
    isInitialized = true;
    % 1) ベースワークスペースから 2D Lookup Table の定義を取得
    xBreakPts = evalin('base','xBreakPts');   % 例: [N1×1] or [1×N1] ベクトル
    yBreakPts = evalin('base','yBreakPts');   % 例: [N2×1] or [1×N2] ベクトル
    z_2DTable = evalin('base','z_2DTable');   % 2D配列, size = [length(yBreakPts), length(xBreakPts)]
 
    % 2) Figureを生成して surf で面を可視化
    figH = figure('Name','2D LUT Debug','Color','w');
    [X, Y] = meshgrid(xBreakPts, yBreakPts);
    surf(X, Y, z_2DTable');  
    colormap('jet');
    shading('interp');
    colorbar;
    hold('on');  % 後で点を重ね描きするので hold on
    xlabel('xBreakPts'); ylabel('yBreakPts'); zlabel('Table Data');
    title('2D Lookup Table Surface');
    % 3) 初期点として plot3 (ここでは初回呼び出し時の x,y,z を描画)
    %    - 出力は Line オブジェクトを受け取って persistent に保存
    lineH = plot3(x, y, z, 'ro', 'MarkerFaceColor','r','MarkerSize',8);
else
    %============================
    % (B) 2回目以降の呼び出し: (x,y,z) の4点を更新する
    %============================
    % ここでは set関数を使わず、直接プロパティ代入で更新
    set(lineH, 'XData', x, 'YData', y, 'ZData', z);
    % lineH.XData = x;
    % lineH.YData = y;
    % lineH.ZData = z;
end
 
% --- 描画の更新 (負荷を抑えるなら 'limitrate' やステップ間引きも検討) ---
drawnow('limitrate');

== matlab function TrajectoryFollowVehicleWith14DoF_/Pack Actor Pose/Cvt2RRSCoodinate ==
  data: pose input; RRSPose output
function RRSPose = convert2RRS(pose)
    RRSPose = pose; %[x, y, yaw, z, pitch, roll]
    RRSPose(3) = pose(3) - 90;
    RRSPose(6) = -pose(5);
    RRSPose(5) = pose(6);
end
